simulink model "Q1S"  (R2022a)
settings: Solver=VariableStepAuto  StartTime=0.0  StopTime=0.5  RelTol=1e-3
settings Model: Creator=Guilherme  LastModifiedBy=Guilherme

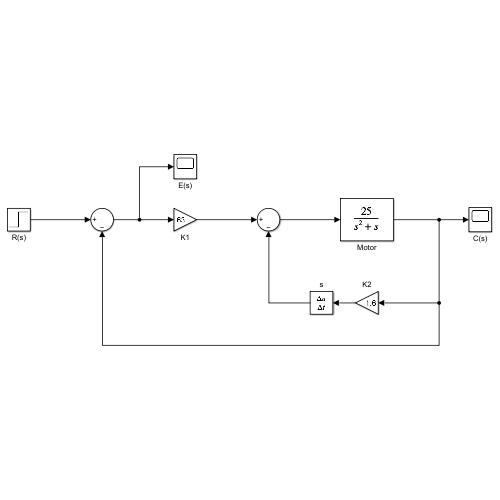
[thumbnail: Simulink's stored preview of the top-level diagram]
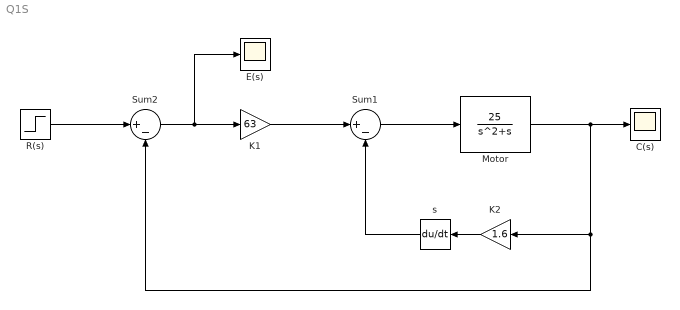
== system Q1S ==
  C(s) : Scope
  E(s) : Scope
  K1 : Gain  Gain=63
  K2 : Gain  Gain=1.6
  Motor : TransferFcn  Numerator=[25]  Denominator=[1 1 0]
  R(s) : Step  Time=0  SampleTime=0
  Sum1 : Sum  Inputs=|+-
  Sum2 : Sum  Inputs=|+-
  s : Derivative
  wires:
  Motor/1 -> K2/1, Sum2/2, C(s)/1
  Sum1/1 -> Motor/1
  K1/1 -> Sum1/1
  K2/1 -> s/1
  Sum2/1 -> K1/1, E(s)/1
  R(s)/1 -> Sum2/1
  s/1 -> Sum1/2
